simulink model "task1-3"  (R2016a)
settings: Solver=VariableStepAuto  StartTime=0.0  StopTime=40.0  RelTol=1e-3
libraries: simulink_extras x5
settings Model: Creator=Misachu  LastModifiedBy=Misachu

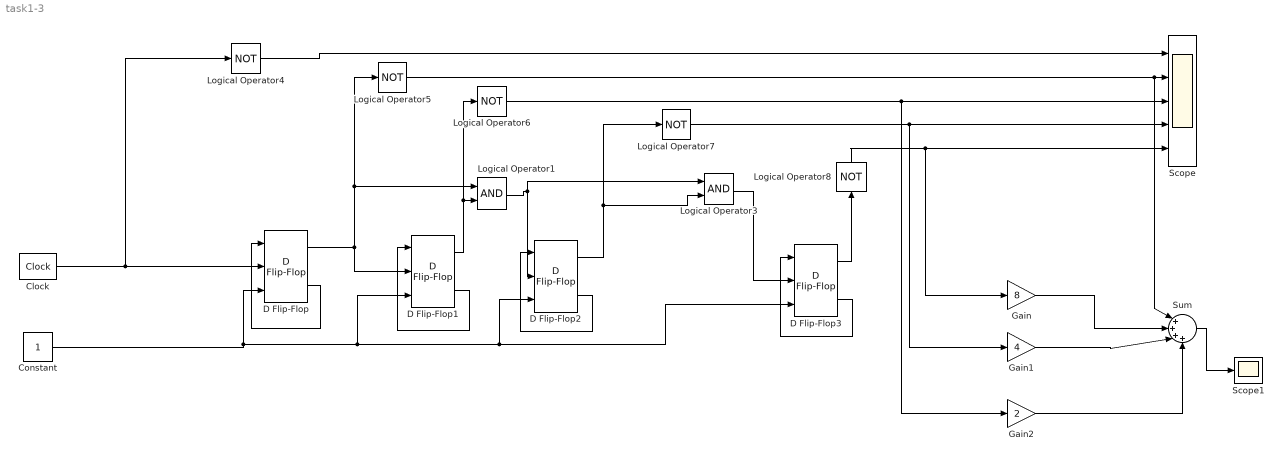
== system task1-3 ==
  Clock : simulink_extras/Flip Flops/Clock  period=2
  Constant : Constant
  D Flip-Flop{,1..3} (4 alike) : simulink_extras/Flip Flops/D Flip-Flop
  Gain : Gain  Gain=8
  Gain1 : Gain  Gain=4
  Gain2 : Gain  Gain=2
  Logical Operator1 : Logic  AllPortsSameDT=off  OutDataTypeStr=boolean
  Logical Operator3 : Logic  AllPortsSameDT=off  OutDataTypeStr=boolean
  Logical Operator{4..8} (5 alike) : Logic  Operator=NOT  AllPortsSameDT=off  OutDataTypeStr=boolean
  Scope : Scope  NumInputPorts=5
  Scope1 : Scope
  Sum : Sum  Inputs=|++++
  wires:
  Clock/1 -> Logical Operator4/1, D Flip-Flop/2
  D Flip-Flop/1 -> Logical Operator5/1, Logical Operator1/1, D Flip-Flop1/2
  D Flip-Flop/2 -> D Flip-Flop/1
  D Flip-Flop1/2 -> D Flip-Flop1/1
  D Flip-Flop2/2 -> D Flip-Flop2/1
  D Flip-Flop3/2 -> D Flip-Flop3/1
  Constant/1 -> D Flip-Flop/3, D Flip-Flop1/3, D Flip-Flop2/3, D Flip-Flop3/3
  D Flip-Flop1/1 -> Logical Operator6/1, Logical Operator1/2
  D Flip-Flop2/1 -> Logical Operator3/2, Logical Operator7/1
  D Flip-Flop3/1 -> Logical Operator8/1
  Logical Operator3/1 -> D Flip-Flop3/2
  Logical Operator1/1 -> Logical Operator3/1, D Flip-Flop2/2
  Gain/1 -> Sum/2
  Gain2/1 -> Sum/4
  Sum/1 -> Scope1/1
  Gain1/1 -> Sum/3
  Logical Operator4/1 -> Scope/1
  Logical Operator5/1 -> Sum/1, Scope/2
  Logical Operator6/1 -> Gain2/1, Scope/3
  Logical Operator7/1 -> Gain1/1, Scope/4
  Logical Operator8/1 -> Gain/1, Scope/5
